simulink model "blockKicker_tSim"  (R2014b)
settings: Solver=ode45  StartTime=0.0  StopTime=160  RelTol=1e-3
settings Model: SnapshotBufferSize=60  SnapshotInterval=1  Creator=Michael  LastModifiedBy=Michael
settings RTWCC: Toolchain=Texas Instruments Code Composer Studio v5 (C2000)

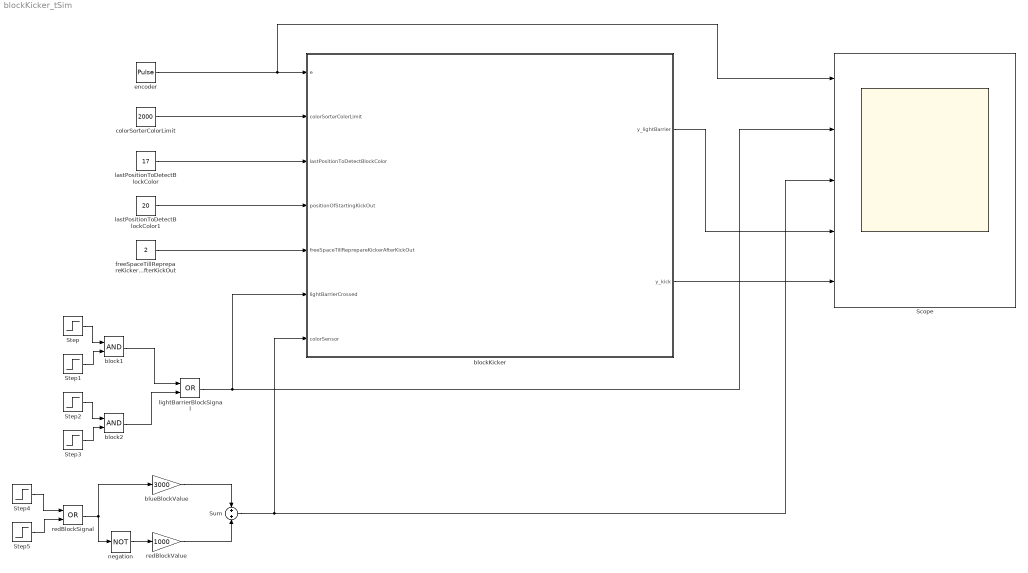
== system blockKicker_tSim ==
  Scope : Scope  NumInputPorts=5
      settings: ShowLegends=on  TimeRange=160  YMin=-3~-2~0~-7~-5  YMax=3~2~4096~7~5
  Step : Step  Time=5  SampleTime=0
  Step1 : Step  Time=15  Before=1  After=0  SampleTime=0
  Step2 : Step  Time=60  SampleTime=0
  Step3 : Step  Time=70  Before=1  After=0  SampleTime=0
  Step4 : Step  Time=75  Before=1  After=0  SampleTime=0
  Step5 : Step  Time=85  SampleTime=0
  Sum : Sum  Inputs=+|+  AccumDataTypeStr=uint16  OutMin=0  OutMax=4095  OutDataTypeStr=uint16
  block1 : Logic  AllPortsSameDT=off  OutDataTypeStr=boolean
  block2 : Logic  AllPortsSameDT=off  OutDataTypeStr=boolean
  blockKicker : Stateflow chart  TreatAsAtomicUnit=on
  blueBlockValue : Gain  Gain=3000  OutMin=0  OutMax=4095  OutDataTypeStr=uint16
  colorSorterColorLimit : Constant  Value=2000  OutMin=0  OutMax=4095  OutDataTypeStr=uint16
  encoder : DiscretePulseGenerator  PulseType=Time based  PulseWidth=50
  freeSpaceTillReprepareKickerAfterKickOut : Constant  Value=2  OutDataTypeStr=uint32
  lastPositionToDetectBlockColor : Constant  Value=17  OutDataTypeStr=uint32
  lastPositionToDetectBlockColor1 : Constant  Value=20  OutDataTypeStr=uint32
  lightBarrierBlockSignal : Logic  Operator=OR  AllPortsSameDT=off  OutDataTypeStr=boolean
  negation : Logic  Operator=NOT  AllPortsSameDT=off  OutDataTypeStr=boolean
  redBlockSignal : Logic  Operator=OR  AllPortsSameDT=off  OutDataTypeStr=boolean
  redBlockValue : Gain  Gain=1000  OutMin=0  OutMax=4095  OutDataTypeStr=uint16
  wires:
  encoder/1 -> Scope/1, blockKicker/1(e)
  Step/1 -> block1/1
  blockKicker/1(y_lightBarrier) -> Scope/4
  blockKicker/2(y_kick) -> Scope/5
  Step1/1 -> block1/2
  lightBarrierBlockSignal/1 -> blockKicker/6(lightBarrierCrossed), Scope/2
  Step2/1 -> block2/1
  Step3/1 -> block2/2
  block1/1 -> lightBarrierBlockSignal/1
  block2/1 -> lightBarrierBlockSignal/2
  Step4/1 -> redBlockSignal/1
  Step5/1 -> redBlockSignal/2
  Sum/1 -> blockKicker/7(colorSensor), Scope/3
  redBlockSignal/1 -> blueBlockValue/1, negation/1
  negation/1 -> redBlockValue/1
  blueBlockValue/1 -> Sum/1
  redBlockValue/1 -> Sum/2
  colorSorterColorLimit/1 -> blockKicker/2(colorSorterColorLimit)
  lastPositionToDetectBlockColor/1 -> blockKicker/3(lastPositionToDetectBlockColor)
  lastPositionToDetectBlockColor1/1 -> blockKicker/4(positionOfStartingKickOut)
  freeSpaceTillReprepareKickerAfterKickOut/1 -> blockKicker/5(freeSpaceTillReprepareKickerAfterKickOut)

== stateflow chart blockKicker_tSim/blockKicker ==
  state lightBarrier_controller [parallel]
    settings: executionOrder=3
    state idle
      entry: y_lightBarrier = int16(0);
    state lightBarrierCrossed
      entry: send(counterFromLightBarrierCrossed.RESET);
      send(color_controller.NEXTBLOCK);
      y_lightBarrier = int16(1);
    (default) -> lightBarrier_controller.idle : /{kicker_controller.enqueuedBlocksToKick =uint8( 0)}
    lightBarrier_controller.idle -> lightBarrierCrossed : [lightBarrierCrossed >= 1]
    lightBarrierCrossed -> lightBarrier_controller.idle : [lightBarrierCrossed <1]
  state counterFromLightBarrierCrossed [parallel]
    settings: executionOrder=1
    state start
      entry: count= uint32(0);
    state highLevel
    state lowLevel
      entry: count = count + 1;
    counterFromLightBarrierCrossed.lowLevel -> counterFromLightBarrierCrossed.highLevel : [e>0]
    (default) -> counterFromLightBarrierCrossed.start
    counterFromLightBarrierCrossed.start -> counterFromLightBarrierCrossed.lowLevel : [e>0]
    counterFromLightBarrierCrossed.highLevel -> counterFromLightBarrierCrossed.lowLevel : [e==0]
    counterFromLightBarrierCrossed -> counterFromLightBarrierCrossed.start : RESET
  state counterFromKick [parallel]
    settings: executionOrder=2
    state start
      entry: count= uint32(0);
    state highLevel
    state lowLevel
      entry: count = count + 1;
    counterFromKick.lowLevel -> counterFromKick.highLevel : [e>0]
    (default) -> counterFromKick.start
    counterFromKick.start -> counterFromKick.lowLevel : [e>0]
    counterFromKick.highLevel -> counterFromKick.lowLevel : [e==0]
    counterFromKick -> counterFromKick.start : RESET
  state kicker_controller [parallel]
    settings: executionOrder=5
    state kick
      entry: send(counterFromKick.RESET);
      enqueuedBlocksToKick = enqueuedBlocksToKick -1;
      y_kick = int16(5);
    state idle
      entry: y_kick = int16(0);
    state reprepareKicker
      entry: y_kick = int16(-5);
    (default) -> kicker_controller.idle
    kicker_controller.idle -> kick : [[counterFromLightBarrierCrossed.count >= positionOfStartingKickOut] && [enqueuedBlocksToKick > 0]]
    reprepareKicker -> kicker_controller.idle
    kick -> reprepareKicker : [counterFromKick.count >= freeSpaceTillReprepareKickerAfterKickOut]
  state color_controller [parallel]
    settings: executionOrder=4
    state blockToKick
      entry: kicker_controller.enqueuedBlocksToKick = kicker_controller.enqueuedBlocksToKick + 1;
    state blockNotToKick
    state waitingForBlockToPassColorSensor
    (default) -> blockNotToKick
    waitingForBlockToPassColorSensor -> (junction 89) [order 1] : [counterFromLightBarrierCrossed.count >= lastPositionToDetectBlockColor]
    (junction 89) -> blockToKick [order 1] : [shouldBeKicked == true]
    blockNotToKick -> waitingForBlockToPassColorSensor : NEXTBLOCK /{shouldBeKicked = true}
    (junction 89) -> (junction 91) [order 2] : [shouldBeKicked == false]
    waitingForBlockToPassColorSensor -> waitingForBlockToPassColorSensor [order 2] : [colorSensor <= colorSorterColorLimit] {shouldBeKicked = false}
    (junction 91) -> blockNotToKick
    blockToKick -> (junction 91)
  data: count local uint32; count local uint32; enqueuedBlocksToKick local uint8 [0..2]; shouldBeKicked local boolean; e input; y_lightBarrier output int16; y_kick output int16; colorSorterColorLimit input uint16 [0..4095]; lastPositionToDetectBlockColor input uint32; positionOfStartingKickOut input uint32; freeSpaceTillReprepareKickerAfterKickOut input uint32; lightBarrierCrossed input; colorSensor input uint16 [0..4095]
  data lastPositionToDetectBlockColor settings: description=length from light barrier to last possible position for color detection of blocks in tics from encoder
  data positionOfStartingKickOut settings: description=length from light barrier to position where kicker starts off kicking out blocks in tics from encoder
  data freeSpaceTillReprepareKickerAfterKickOut settings: description=space to wait after the kick out of a block till kicker reprepares (crosses the drive lane again) in tics from encoder
  events: RESET local FUNCTION_CALL_EVENT; RESET local FUNCTION_CALL_EVENT; NEXTBLOCK local FUNCTION_CALL_EVENT
